simulink model "myModel1"  (R2021a)
settings: Solver=FixedStepAuto  StartTime=0.0  StopTime=10.0  RelTol=1e-3
settings Model: Creator=ppatil  LastModifiedBy=ppatil
settings SolverCC: AlgebraicLoopSolver=TrustRegion
settings DebuggingCC: SFMachineParentedDataDiag=warning

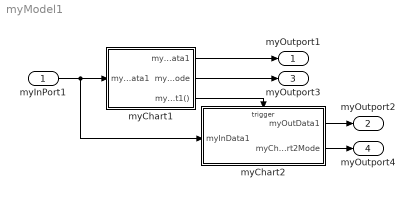
== system myModel1 ==
  myInPort1 : Inport
  myChart1 : Stateflow chart  TreatAsAtomicUnit=on
  myChart2 : Stateflow chart  TreatAsAtomicUnit=on
  myOutport1 : Outport
  myOutport2 : Outport  Port=2
  myOutport3 : Outport  Port=3
  myOutport4 : Outport  Port=4
  wires:
  myChart1/1(myOutData1) -> myOutport1/1
  myInPort1/1 -> myChart2/1(myInData1), myChart1/1(myInData1)
  myChart1/3(myEvent1()) -> myChart2/Trigger
  myChart2/1(myOutData1) -> myOutport2/1
  myChart1/2(myChart1Mode) -> myOutport3/1
  myChart2/2(myChart2Mode) -> myOutport4/1

== stateflow chart myModel1/myChart2 ==
  state myState2
    myOutData1=myMfcn1(myInData1);
  state myState1
    myOutData1=myGfcn1(myInData1);
  state myGfcn1_OutArg1=myGfcn1(myGfcn1_InArg1) [function]
    (default) -> (junction 16) [order 1] : [myGfcn1_InArg1>2]{myGfcn1_OutArg1=myGfcn1_InArg1+1;}
    (default) -> (junction 16) [order 2] : {myGfcn1_OutArg1=myGfcn1_InArg1+2;}
  state myState3
    myOutData1=342;
  (default) -> myState1
  myState1 -> (junction 4)
  (junction 4) -> myState2 [order 1] : [myInData1==487]
  (junction 4) -> myState3 [order 2] : [myInData1==488]
  data: myGfcn1_InArg1 function_input; myGfcn1_OutArg1 function_output; myMfcn1_InArg1 function_input; myMfcn1_OutArg1 function_output; myInData1 input; myOutData1 output; myChart2Mode output Enum: myChart2ModeType
  events: myInEvent1 input FUNCTION_CALL_EVENT
  function myMfcn1_OutArg1=myMfcn1(myMfcn1_InArg1):
    | function myMfcn1_OutArg1=myMfcn1(myMfcn1_InArg1)
    |     if myMfcn1_InArg1 > 3
    |         myMfcn1_OutArg1=myMfcn1_InArg1+1;
    |     else
    |         myMfcn1_OutArg1=myMfcn1_InArg1+2;
    |     end
    | end

== stateflow chart myModel1/myChart1 ==
  state myState1
    myOutData1=myGfcn1(myInData1);
    du:
    send(myEvent1);
  state myState2
    myOutData1=myMfcn1(myInData1);
  state myGfcn1_OutArg1=myGfcn1(myGfcn1_InArg1) [function]
    (default) -> (junction 29) [order 1] : [myGfcn1_InArg1>2]{myGfcn1_OutArg1=myGfcn1_InArg1+1;}
    (default) -> (junction 29) [order 2] : {myGfcn1_OutArg1=myGfcn1_InArg1+myMachineData1;}
  state myState3
    myOutData1=342;
  (default) -> myState1
  myState1 -> (junction 4)
  (junction 4) -> myState2 [order 1] : [myInData1==487]
  (junction 4) -> myState3 [order 2] : [myInData1==488]
  data: myGfcn1_InArg1 function_input; myGfcn1_OutArg1 function_output; myMfcn1_InArg1 function_input; myMfcn1_OutArg1 function_output; myInData1 input; myOutData1 output; myChart1Mode output Enum: myChart1ModeType
  events: myEvent1 output FUNCTION_CALL_EVENT
  function myMfcn1_OutArg1=myMfcn1(myMfcn1_InArg1):
    | function myMfcn1_OutArg1=myMfcn1(myMfcn1_InArg1)
    |     if myMfcn1_InArg1 > 3
    |         myMfcn1_OutArg1=myMfcn1_InArg1+1;
    |     else
    |         myMfcn1_OutArg1=myMfcn1_InArg1+2;
    |     end
    | end
